simulink model "IIR_Simulink"  (R2020a)
settings: Solver=VariableStepAuto  StartTime=0.0  StopTime=Inf  RelTol=1e-3
libraries: dspsnks4 x1, dspvision x1, simulink x1
settings Model: Creator=Michele  LastModifiedBy=miche
settings DataIOCC: ReturnWorkspaceOutputs=off
settings DebuggingCC: ArithmeticOperatorsInVariantConditions=warning
settings SFSimCC: SimUseLocalCustomCode=off  CustomCodeUndefinedFunction=UseInterfaceOnly
settings RTWCC: RTWUseLocalCustomCode=off
settings CodeAppCC: StateflowObjectComments=on

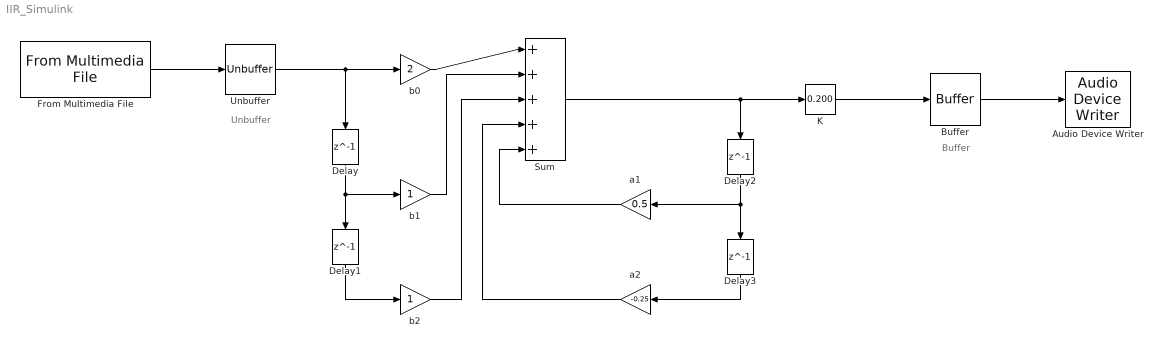
== system IIR_Simulink ==
  note: Buffer
  note: Unbuffer
  Audio Device Writer : dspsnks4/Audio Device Writer  Driver=DirectSound  Device=Default  InheritSampleRate=on  SampleRate=44100  BitDepth=16-bit integer  BufferSize=4096  NumBuffers=10  DefaultOutputChannelMapping=on  OutputChannelMapping=1:2  OutputNumUnderrunSamples=off  DriverIdx=1  DeviceWarnFlag=''
  Buffer : Buffer  N=1024  OutputFrames=off
  Delay{,1..3} (4 alike) : Delay  DelayLength=1
  From Multimedia File : dspvision/From Multimedia File  inputFilename=C:\Users\miche\Documents\MATLAB\audio.wav  readRange=[1 Inf]  loop=on  numPlays=inf  outputStreams=Audio only  videoDataType=single  audioDataType=double  inheritSampleTime=on  userDefinedSampleTime=1/30  noAudioOutput=off  isIntensityVideo=off  fourcc=RGB  colorVideoFormat=Separate color signals  outputEOF=off  dataOrg=Column-major  audioFrameSize=1024  computeAudioFrameSize=off  outSamplingMode=Sample based
  K : simulink/Math Operations/Slider Gain  gain=0.200  low=0  high=2
  Sum : Sum  Inputs=|+++++
  Unbuffer : Unbuffer
  a1 : Gain  Gain=0.5  OutDataTypeStr=double
  a2 : Gain  Gain=-0.25  OutDataTypeStr=double
  b0 : Gain  Gain=2  OutDataTypeStr=double
  b1 : Gain  OutDataTypeStr=double
  b2 : Gain  OutDataTypeStr=double
  wires:
  Unbuffer/1 -> Delay/1, b0/1
  b0/1 -> Sum/1
  Delay/1 -> b1/1, Delay1/1
  Delay1/1 -> b2/1
  Delay2/1 -> Delay3/1, a1/1
  Delay3/1 -> a2/1
  Sum/1 -> K/1, Delay2/1
  b1/1 -> Sum/2
  b2/1 -> Sum/3
  a2/1 -> Sum/4
  a1/1 -> Sum/5
  K/1 -> Buffer/1
  From Multimedia File/1 -> Unbuffer/1
  Buffer/1 -> Audio Device Writer/1
